simulink model "AceleracionImu"  (R2022b)
settings: Solver=VariableStepAuto  StartTime=0.0  StopTime=6  RelTol=1e-3
libraries: dsparch4 x3, simulink x1
settings Model: Creator=mique  LastModifiedBy=mique
settings DataIOCC: ReturnWorkspaceOutputs=off

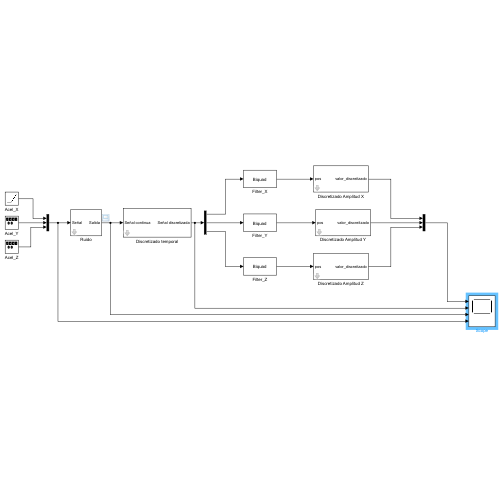
[thumbnail: Simulink's stored preview of the top-level diagram]
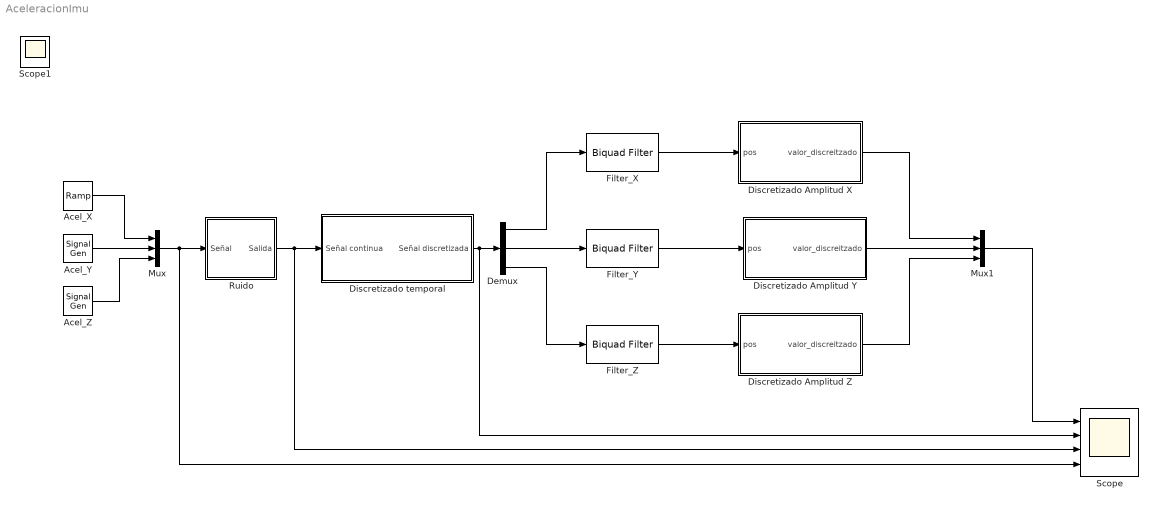
== system AceleracionImu ==
  Acel_X : simulink/Sources/Ramp  slope=1  start=0  InitialOutput=0
  Acel_Y : SignalGenerator  WaveForm=sawtooth  Frequency=2
  Acel_Z : SignalGenerator  Amplitude=3
  Demux : Demux  Outputs=3
  Discretizado Amplitud X : Subsystem  mask{Num_Val=70, Max=10, Min=0}
      mask prompts: Num_Val "Numero de valores distintos"; Max "Maximo valor"; Min "Minimo valor"
  Discretizado Amplitud Y : Subsystem  mask{Num_Val=200, Max=2, Min=-2}
      mask prompts: Num_Val "Numero de valores distintos"; Max "Maximo valor"; Min "Minimo valor"
  Discretizado Amplitud Z : Subsystem  mask{Num_Val=40, Max=3.7, Min=-3.7}
      mask prompts: Num_Val "Numero de valores distintos"; Max "Maximo valor"; Min "Minimo valor"
  Discretizado temporal : Subsystem  mask{Tiempo_Discretizado=0.0005}
      mask prompts: Tiempo_Discretizado "Tiempo de discretizacion (s)"
      mask DialogControl DescGroupVar Prompt: Discretiza una señal mediante un ZOH con un tiempo definido
  Filter_X : dsparch4/Biquad Filter  Tag=BlockMethodSubSystem  FilterSource=Dialog parameters  CoeffSource=Specify via dialog  FilterObject=BQF  IIRFiltStruct=Direct form II  BiQuadCoeffs=[1 2 1 1 -1.56101807580071816 0.641351538057563175]  ScaleValues=[0.0200833655642112356;1]  IC=0  ICnum=0  ICden=0  a0Flag=Warning  optimizeScaleValues=on  ScaleValueMode=Specify via input port (g)  InputProcessing=Columns as channels (frame based)  roundingMode=Floor  overflowMode=off  scaleValueFracLength=14  denProdOutputFracLength=30  denAccumFracLength=30  secondMemoryFracLength=15
  Filter_Y : dsparch4/Biquad Filter  Tag=BlockMethodSubSystem  FilterSource=Dialog parameters  CoeffSource=Specify via dialog  FilterObject=BQF  IIRFiltStruct=Direct form II  BiQuadCoeffs=[1 2 1 1 -1.73631016553472994 0.825664548620660854;1 2 1 1 -1.52169042607224592 0.6000000000000002;1 1 0 1 -0.72654252800536101 0]  ScaleValues=[0.0223385957714827763;0.0195773934819385709;0.13672873599731955;1]  IC=0  ICnum=0  ICden=0  a0Flag=Warning  optimizeScaleValues=on  ScaleValueMode=Specify via input port (g)  InputProcessing=Columns as channels (frame based)  roundingMode=Floor  overflowMode=off  scaleValueFracLength=14  denProdOutputFracLength=30  denAccumFracLength=30  secondMemoryFracLength=15
  Filter_Z : dsparch4/Biquad Filter  Tag=BlockMethodSubSystem  FilterSource=Dialog parameters  CoeffSource=Specify via dialog  FilterObject=BQF  IIRFiltStruct=Direct form II  BiQuadCoeffs=[1 2 1 1 -1.73631016553472994 0.825664548620660854;1 2 1 1 -1.52169042607224592 0.6000000000000002;1 1 0 1 -0.72654252800536101 0]  ScaleValues=[0.0223385957714827763;0.0195773934819385709;0.13672873599731955;1]  IC=0  ICnum=0  ICden=0  a0Flag=Warning  optimizeScaleValues=on  ScaleValueMode=Specify via input port (g)  InputProcessing=Columns as channels (frame based)  roundingMode=Floor  overflowMode=off  scaleValueFracLength=14  denProdOutputFracLength=30  denAccumFracLength=30  secondMemoryFracLength=15
  Mux : Mux  Inputs=3
  Mux1 : Mux  Inputs=3
  Ruido : Subsystem  mask{M=0, V=0.005, f=1000}
      mask prompts: M "Media"; V "Varianza"; f "Frecuencia (Hz)"
      mask init:
      | T=1/f;
      mask DialogControl DescGroupVar Prompt: Añadidor de Ruido
      mask DialogControl DescTextVar Prompt: Añade un ruido blanco Gausiano con los siguientes valores:
  Scope : Scope  NumInputPorts=4
  Scope1 : Scope
  wires:
  Acel_Y/1 -> Mux/2
  Acel_X/1 -> Mux/1
  Acel_Z/1 -> Mux/3
  Demux/1 -> Filter_X/1
  Demux/3 -> Filter_Z/1
  Filter_X/1 -> Discretizado Amplitud X/1(pos)
  Filter_Z/1 -> Discretizado Amplitud Z/1(pos)
  Discretizado Amplitud X/1(valor_discreitzado) -> Mux1/1
  Mux/1 -> Scope/4, Ruido/1(Señal)
  Discretizado Amplitud Z/1(valor_discreitzado) -> Mux1/3
  Mux1/1 -> Scope/1
  Discretizado temporal/1(Señal discretizada) -> Scope/2, Demux/1
  Ruido/1(Salida) -> Scope/3, Discretizado temporal/1(Señal continua)
  Discretizado Amplitud Y/1(valor_discreitzado) -> Mux1/2
  Filter_Y/1 -> Discretizado Amplitud Y/1(pos)
  Demux/2 -> Filter_Y/1

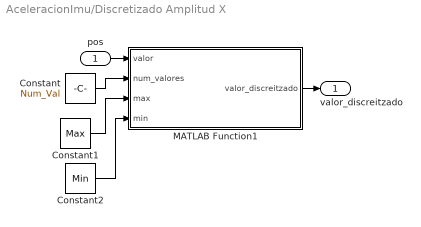
== system AceleracionImu/Discretizado Amplitud X ==
  pos : Inport
  Constant : Constant  Value=Num_Val
  Constant1 : Constant  Value=Max
  Constant2 : Constant  Value=Min
  MATLAB Function1 : MATLAB Function  TreatAsAtomicUnit=on
  valor_discreitzado : Outport
  wires:
  MATLAB Function1/1(valor_discreitzado) -> valor_discreitzado/1
  Constant1/1 -> MATLAB Function1/3(max)
  Constant/1 -> MATLAB Function1/2(num_valores)
  Constant2/1 -> MATLAB Function1/4(min)
  pos/1 -> MATLAB Function1/1(valor)

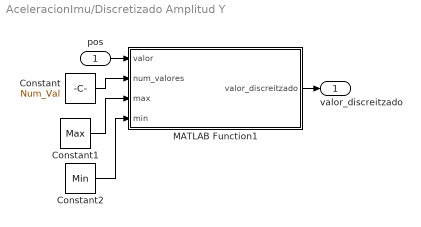
== system AceleracionImu/Discretizado Amplitud Y ==
  pos : Inport
  Constant : Constant  Value=Num_Val
  Constant1 : Constant  Value=Max
  Constant2 : Constant  Value=Min
  MATLAB Function1 : MATLAB Function  TreatAsAtomicUnit=on
  valor_discreitzado : Outport
  wires:
  pos/1 -> MATLAB Function1/1(valor)
  Constant2/1 -> MATLAB Function1/4(min)
  Constant/1 -> MATLAB Function1/2(num_valores)
  Constant1/1 -> MATLAB Function1/3(max)
  MATLAB Function1/1(valor_discreitzado) -> valor_discreitzado/1

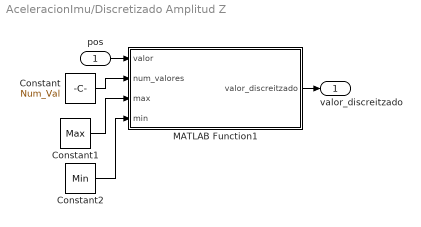
== system AceleracionImu/Discretizado Amplitud Z ==
  pos : Inport
  Constant : Constant  Value=Num_Val
  Constant1 : Constant  Value=Max
  Constant2 : Constant  Value=Min
  MATLAB Function1 : MATLAB Function  TreatAsAtomicUnit=on
  valor_discreitzado : Outport
  wires:
  MATLAB Function1/1(valor_discreitzado) -> valor_discreitzado/1
  Constant1/1 -> MATLAB Function1/3(max)
  Constant/1 -> MATLAB Function1/2(num_valores)
  Constant2/1 -> MATLAB Function1/4(min)
  pos/1 -> MATLAB Function1/1(valor)

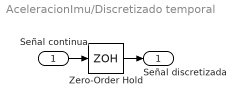
== system AceleracionImu/Discretizado temporal ==
  Señal continua : Inport
  Zero-Order Hold : ZeroOrderHold  SampleTime=Tiempo_Discretizado
  Señal discretizada : Outport
  wires:
  Zero-Order Hold/1 -> Señal discretizada/1
  Señal continua/1 -> Zero-Order Hold/1

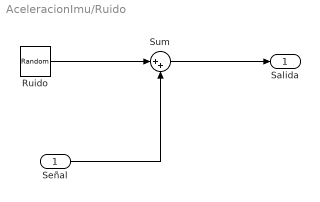
== system AceleracionImu/Ruido ==
  Señal : Inport
  Ruido : RandomNumber  Mean=M  Variance=V  Seed=10  SampleTime=T
  Sum : Sum  Inputs=|++
  Salida : Outport
  wires:
  Sum/1 -> Salida/1
  Ruido/1 -> Sum/1
  Señal/1 -> Sum/2

== matlab function AceleracionImu/Discretizado Amplitud Y/MATLAB Function1 ==
  data: valor input; valor_discreitzado output; num_valores input; max input; min input
function valor_discreitzado  = fcn(valor,num_valores,max,min)

if(valor>max)
    valor_discreitzado=max;
    return
end
if(valor<min)
    valor_discreitzado=min;
    return
end


valor_escalon=(max-min)/(num_valores-1);


i=min;
 while(i<max)
    if(i+valor_escalon/2>valor)
        valor_discreitzado=i;
        return
    end
    i=i+valor_escalon;
end



      valor_discreitzado=max;
end

== matlab function AceleracionImu/Discretizado Amplitud Z/MATLAB Function1 ==
  data: valor input; valor_discreitzado output; num_valores input; max input; min input
function valor_discreitzado  = fcn(valor,num_valores,max,min)

if(valor>max)
    valor_discreitzado=max;
    return
end
if(valor<min)
    valor_discreitzado=min;
    return
end


valor_escalon=(max-min)/(num_valores-1);


i=min;
 while(i<max)
    if(i+valor_escalon/2>valor)
        valor_discreitzado=i;
        return
    end
    i=i+valor_escalon;
end



      valor_discreitzado=max;
end

== matlab function AceleracionImu/Discretizado Amplitud X/MATLAB Function1 ==
  data: valor input; valor_discreitzado output; num_valores input; max input; min input
function valor_discreitzado  = fcn(valor,num_valores,max,min)

if(valor>max)
    valor_discreitzado=max;
    return
end
if(valor<min)
    valor_discreitzado=min;
    return
end


valor_escalon=(max-min)/(num_valores-1);


i=min;
 while(i<max)
    if(i+valor_escalon/2>valor)
        valor_discreitzado=i;
        return
    end
    i=i+valor_escalon;
end



      valor_discreitzado=max;
end
